simulink model "blockDiagram"  (R2025a)
settings: Solver=VariableStepAuto  StartTime=0.0  StopTime=500  RelTol=1e-3
model workspace (MAT data in the model file):
  C_V = 1.1e-06
  I0 = 0.124
  J = 6.3e-06
  K_E = 0.006741
  K_M = 0.0644
  L = 0.000238
  R = 3.23
  U_N = 36
  n0 = 5500
libraries: simulink x1
settings Model: Creator=josef  LastModifiedBy=aladdin

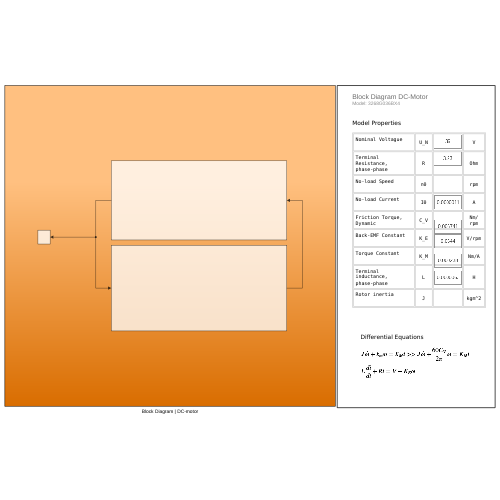
[thumbnail: Simulink's stored preview of the top-level diagram]
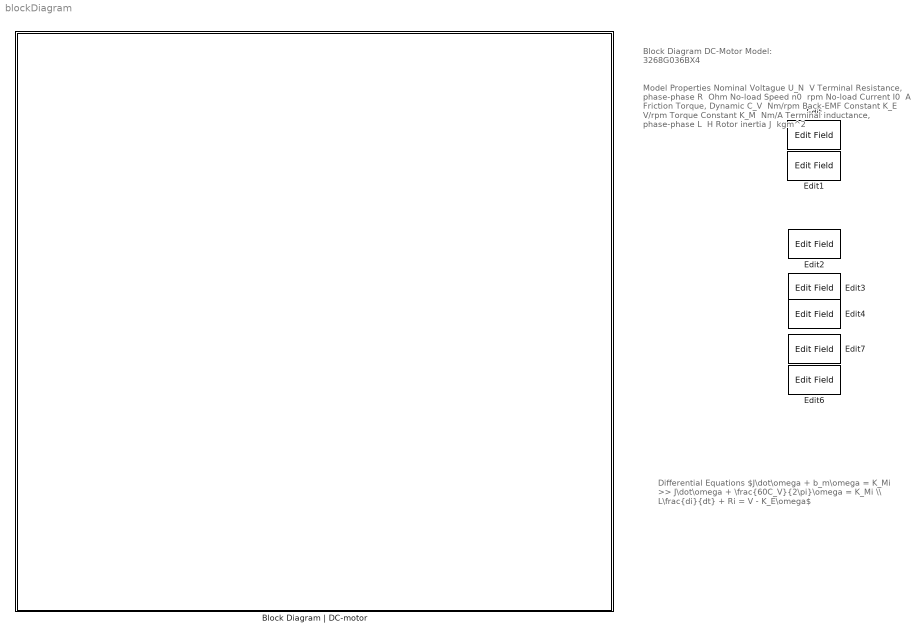
== system blockDiagram ==
  note: Differential Equations
      |
      | $J\dot\omega + b_m\omega = K_Mi >> J\dot\omega + \frac{60C_V}{2\pi}\omega = K_Mi \\ L\frac{di}{dt} + Ri = V - K_E\omega$
  note: Model Properties
      |
      | Nominal Voltague
      |
      | U_N
      | ​
      | V
      |
      | Terminal Resistance,
      | phase-phase
      | R
      | ​
      | Ohm
      |
      | No-load Speed
      |
      | n0
      | ​
      | rpm
      |
      | No-load Current
      |
      | I0
      | ​
      | A
      |
      | Friction Torque,
      | Dynamic
      | C_V
      | ​
      | Nm/rpm
      |
      | Back-EMF Constant
      |
      | K_E
      | ​
      | V/rpm
      |
      | Torque Constant
      |
      | K_M
      | ​
      | Nm/A
      |
      | Terminal inductance,
      | phase-phase
      | L
      | ​
      | H
      |
      | Rotor inertia
      |
      | J
      | ​
      | kgm^2
  note: Block Diagram DC-Motor
      | Model: 3268G036BX4
  Block Diagram | DC-motor : Subsystem
  Edit{,1..4,6..7} (7 alike) : EditField  LabelPosition=Hide  ShowInitialText=on  Alignment=Center  Opacity=0

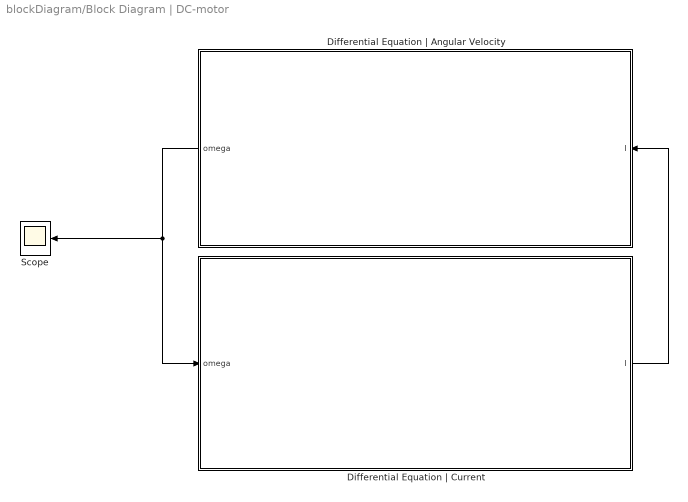
== system blockDiagram/Block Diagram | DC-motor ==
  Differential Equation | Angular Velocity : Subsystem
  Differential Equation | Current : Subsystem
  Scope : Scope
      settings: ActiveDisplayYMinimum=4336.4939458036024  ActiveDisplayYMaximum=6133.1035324379054
  wires:
  Differential Equation | Current/1(I) -> Differential Equation | Angular Velocity/1(I)
  Differential Equation | Angular Velocity/1(omega) -> Differential Equation | Current/1(omega), Scope/1

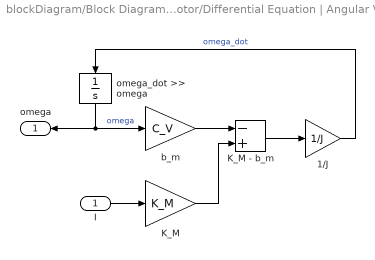
== system blockDiagram/Block Diagram | DC-motor/Differential Equation | Angular Velocity ==
  I : Inport
  1/J : Gain  Gain=1/J
  K_M : Gain  Gain=K_M
  K_M - b_m : Sum  Inputs=-+
  b_m : Gain  Gain=C_V
  omega_dot >> omega : Integrator
  omega : Outport
  wires:
  b_m/1 -> K_M - b_m/1
  omega_dot >> omega/1 -> omega/1, b_m/1  "omega"
  K_M/1 -> K_M - b_m/2
  I/1 -> K_M/1
  1/J/1 -> omega_dot >> omega/1  "omega_dot"
  K_M - b_m/1 -> 1/J/1

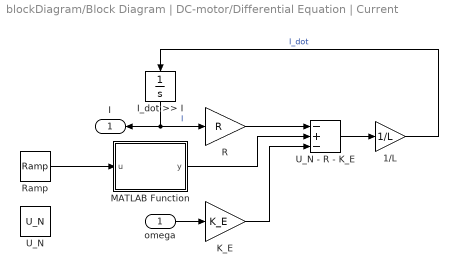
== system blockDiagram/Block Diagram | DC-motor/Differential Equation | Current ==
  omega : Inport
  1/L : Gain  Gain=1/L
  I_dot >> I : Integrator
  K_E : Gain  Gain=K_E
  MATLAB Function : MATLAB Function  TreatAsAtomicUnit=on
  R : Gain  Gain=R
  Ramp : simulink/Sources/Ramp  slope=1  start=0  InitialOutput=0
  U_N : Constant  Value=U_N
  U_N - R - K_E : Sum  Inputs=-+-
  I : Outport
  wires:
  I_dot >> I/1 -> R/1, I/1  "I"
  K_E/1 -> U_N - R - K_E/3
  U_N - R - K_E/1 -> 1/L/1
  omega/1 -> K_E/1
  R/1 -> U_N - R - K_E/1
  1/L/1 -> I_dot >> I/1  "I_dot"
  Ramp/1 -> MATLAB Function/1(u)
  MATLAB Function/1(y) -> U_N - R - K_E/2

== matlab function blockDiagram/Block Diagram | DC-motor/Differential Equation | Current/MATLAB Function ==
  data: u input; y output
function y = fcn(u)

    if (u < 180)
        z = 0.2 * u;

    elseif u >= 480
        z = 36-(0.2 * (u-480));
        if z < 0
            z = 0;
        end
    else
        z = 36;
    end

y = z;
